simulink model "gm_sampleModel1802_5_sub"  (R2023a)
settings: Solver=VariableStepAuto  StartTime=0.0  StopTime=10.0  RelTol=1e-3
libraries: simulink x1
settings Model: Creator=user1  LastModifiedBy=user1
settings OptimizationCC: BlockReduction=off  ConditionallyExecuteInputs=off
settings DebuggingCC: InheritedTsInSrcMsg=none

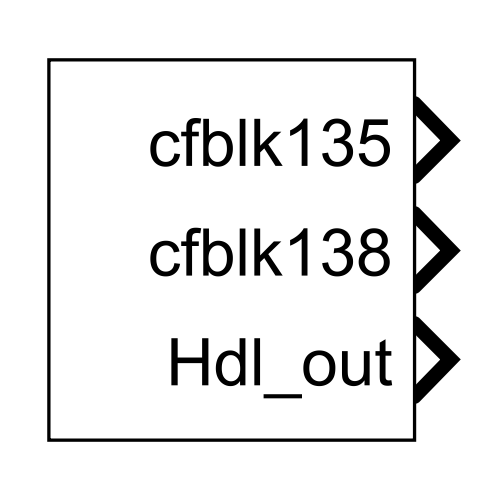
[thumbnail: Simulink's stored preview of the top-level diagram]
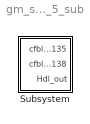
== system gm_sampleModel1802_5_sub ==
  Subsystem : Subsystem

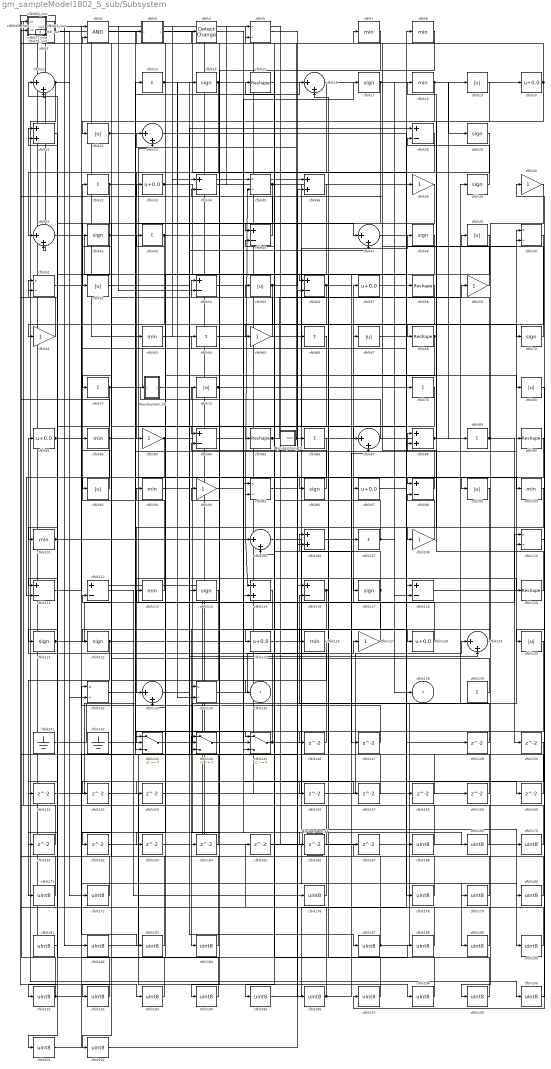
== system gm_sampleModel1802_5_sub/Subsystem ==
  Mysubsystem_19 : Subsystem
  Mysubsystem_30 : Subsystem
  Mysubsystem_45 : Subsystem
  cfblk1 : Subsystem  mask(Compare To Zero){relop=<=, OutDataTypeStr=uint8, ZeroCross=on}
      mask prompts: relop "Simulink:masks:Operator_MP"; OutDataTypeStr "Simulink:masks:OutputDataType_MP"; ZeroCross "Simulink:masks:EnableZerocrossingDetection_MP"
      mask help: Simulink:masks:CompareToZero_MD
      mask init:
      | OutDataTypeStr = 'uint8';
      | ZeroCross = 'on';
      | blkName = 'sampleModel1802_5_sub/Subsystem/cfblk1';
      | relop = '<=';
      | setValue = 'fixdt(0, 8)';
      mask TypeOptions relop: == | ~= | < | <= | >= | >
      mask TypeOptions OutDataTypeStr: Simulink:masks:uint8 | Simulink:masks:boolean
      mask Callback ZeroCross: sl('zeroCrossEnable', gcbh);
      mask Display: disp([relop,' 0'])
  cfblk{7..8,18,63,82,93,100..101,113,126} (10 alike) : MinMax  OutDataTypeStr=uint8
  cfblk103_inst : Subsystem
  cfblk{11,16,23,41,47,87,105,129,133} (9 alike) : Sum  Inputs=|++  OutDataTypeStr=uint8
  cfblk{21,36,88,106,115} (5 alike) : Sum  OutDataTypeStr=uint8
  cfblk{13,32,43,64,66,72,78,86,89,107} (10 alike) : Sum  Inputs=+  OutDataTypeStr=uint8
  cfblk{38,40,59,61,65,83,94,108,127} (9 alike) : Gain  OutDataTypeStr=uint8
  cfblk{5,35,50..51,95,110,132,134} (8 alike) : Product  Inputs=*/  OutDataTypeStr=uint8  RndMeth=Zero  SaturateOnIntegerOverflow=on
  cfblk{28,34,45,54,56,84,98,111..112,116,118} (11 alike) : Sum  Inputs=+-  OutDataTypeStr=uint8
  cfblk{14,17,29,39,42,48,70,96,114,117,121..122} (12 alike) : Signum
  cfblk{15,58,68,85,90,120} (6 alike) : Reshape
  cfblk{20,33,57,81,97,125,128} (7 alike) : Bias  Bias=0.0  SaturateOnIntegerOverflow=off
  cfblk{19,22,49,52,55,67,74,80,92,99,130} (11 alike) : Abs  OutDataTypeStr=uint8  SaturateOnIntegerOverflow=off
  cfblk131_inst : Subsystem
  cfblk139 : Constant  OutDataTypeStr=uint8  SampleTime=-1
  cfblk141 : Ground
  cfblk142 : Ground
  cfblk143 : Switch  OutDataTypeStr=uint8  SaturateOnIntegerOverflow=off  InputSameDT=off
  cfblk144 : Switch  OutDataTypeStr=uint8  SaturateOnIntegerOverflow=off  InputSameDT=off
  cfblk145 : Switch  OutDataTypeStr=uint8  SaturateOnIntegerOverflow=off  InputSameDT=off
  cfblk{146..147,149..153,156..167} (19 alike) : Delay  SampleTime=1
  cfblk{168..172,176,178..184,187..202} (29 alike) : DataTypeConversion  OutDataTypeStr=uint8  SaturateOnIntegerOverflow=off  RndMeth=Floor
  cfblk2 : Logic  AllPortsSameDT=off  OutDataTypeStr=boolean
  cfblk24_inst : Subsystem
  cfblk25_inst : Subsystem
  cfblk3 : Subsystem  mask(Compare To Constant){relop=<=, const=double(3), OutDataTypeStr=uint8, ZeroCross=on}
      mask prompts: relop "Simulink:masks:Operator_MP"; const "Simulink:masks:ConstantValue_MP"; OutDataTypeStr "Simulink:masks:OutputDataType_MP"; ZeroCross "Simulink:masks:EnableZerocrossingDetection_MP"
      mask help: Simulink:masks:CompareToConstant_MD
      mask init:
      | OutDataTypeStr = 'uint8';
      | ZeroCross = 'on';
      | blkName = 'sampleModel1802_5_sub/Subsystem/cfblk3';
      | const = double(3);
      | const_str = '3.0';
      | const_val = double(3);
      | relop = '<=';
      | setValue = 'fixdt(0, 8)';
      | str = '<= 3';
      mask TypeOptions relop: == | ~= | < | <= | >= | >
      mask TypeOptions OutDataTypeStr: Simulink:masks:uint8 | Simulink:masks:boolean
      mask Callback ZeroCross: sl('zeroCrossEnable', gcbh);
      mask Display: disp(str)
  cfblk4 : simulink/Logic and Bit Operations/Detect Change  vinit=0  OutDataTypeStr=uint8
      settings: LibrarySourceBlock=|
      | hdlsllib/Logic and Bit
      | Operations/Detect
      | Change
  cfblk53_inst : Subsystem
  cfblk60_inst : Subsystem
  cfblk69_inst : Subsystem
  cfblk71_inst : Subsystem
  cfblk75_inst : Subsystem
  cfblk135 : Outport  OutDataTypeStr=uint8  SampleTime=1  VectorParamsAs1DForOutWhenUnconnected=off
  cfblk138 : Outport  Port=2  OutDataTypeStr=uint8  SampleTime=1  VectorParamsAs1DForOutWhenUnconnected=off
  Hdl_out : Outport  Port=3  OutDataTypeStr=uint8
  wires:
  Mysubsystem_19/1(Out1) -> cfblk25_inst/1(in1), cfblk23/1
  Mysubsystem_30/1(Out1) -> Mysubsystem_45/1(In1)
  Mysubsystem_45/1(Out1) -> cfblk112/1
  cfblk1/1(y) -> cfblk193/1, cfblk172/1
  cfblk100/1 -> cfblk133/1
  cfblk101/1 -> cfblk115/1, cfblk35/2
  cfblk103_inst/1(out1) -> cfblk182/1
  cfblk105/1 -> cfblk190/1
  cfblk106/1 -> cfblk57/1
  cfblk107/1 -> cfblk15/1, cfblk138/1
  cfblk108/1 -> cfblk98/2
  cfblk11/1 -> cfblk200/1, cfblk132/2
  cfblk110/1 -> cfblk197/1
  cfblk111/1 -> cfblk64/1
  cfblk112/1 -> cfblk176/1
  cfblk113/1 -> cfblk32/1
  cfblk114/1 -> cfblk202/1
  cfblk115/1 -> cfblk162/1
  cfblk116/1 -> cfblk16/2, cfblk125/1
  cfblk117/1 -> cfblk74/1, cfblk184/1
  cfblk118/1 -> cfblk50/1
  cfblk120/1 -> cfblk88/1
  cfblk121/1 -> cfblk97/1, cfblk23/2
  cfblk122/1 -> cfblk171/1, cfblk17/1
  cfblk125/1 -> cfblk48/1
  cfblk126/1 -> cfblk134/1
  cfblk127/1 -> cfblk54/1
  cfblk128/1 -> cfblk113/1
  cfblk129/1 -> cfblk122/1
  cfblk13/1 -> cfblk114/1, cfblk134/2
  cfblk130/1 -> cfblk143/2
  cfblk131_inst/1(out1) -> cfblk89/1
  cfblk132/1 -> cfblk145/1
  cfblk133/1 -> cfblk129/2
  cfblk134/1 -> cfblk127/1
  cfblk139/1 -> cfblk82/1
  cfblk14/1 -> cfblk68/1, cfblk83/1, cfblk164/1
  cfblk141/1 -> cfblk90/1
  cfblk142/1 -> cfblk13/1
  cfblk143/1 -> cfblk110/2
  cfblk144/1 -> cfblk88/2
  cfblk145/1 -> cfblk81/1, cfblk107/1
  cfblk146/1 -> cfblk11/1
  cfblk147/1 -> cfblk132/1
  cfblk149/1 -> cfblk116/2
  cfblk15/1 -> cfblk45/1
  cfblk150/1 -> cfblk192/1
  cfblk151/1 -> cfblk16/1
  cfblk152/1 -> cfblk198/1
  cfblk153/1 -> cfblk110/1
  cfblk156/1 -> cfblk129/1
  cfblk157/1 -> cfblk133/2
  cfblk158/1 -> cfblk144/1
  cfblk159/1 -> cfblk45/2
  cfblk16/1 -> cfblk85/1
  cfblk160/1 -> cfblk2/2
  cfblk161/1 -> cfblk69_inst/2(in2)
  cfblk162/1 -> cfblk34/1
  cfblk163/1 -> cfblk180/1
  cfblk164/1 -> cfblk131_inst/2(in2)
  cfblk165/1 -> cfblk189/1
  cfblk166/1 -> cfblk24_inst/2(in2)
  cfblk167/1 -> cfblk1/1(u)
  cfblk168/1 -> cfblk55/1
  cfblk169/1 -> cfblk3/1(u)
  cfblk17/1 -> cfblk121/1, cfblk118/2
  cfblk170/1 -> cfblk94/1
  cfblk171/1 -> cfblk60_inst/1(in1)
  cfblk172/1 -> cfblk60_inst/2(in2)
  cfblk176/1 -> cfblk25_inst/2(in2)
  cfblk178/1 -> cfblk112/2
  cfblk179/1 -> cfblk24_inst/1(in1)
  cfblk18/1 -> cfblk29/1, cfblk105/2
  cfblk180/1 -> cfblk51/1
  cfblk181/1 -> cfblk51/2
  cfblk182/1 -> cfblk116/1
  cfblk183/1 -> cfblk103_inst/1(in1)
  cfblk184/1 -> cfblk103_inst/2(in2)
  cfblk187/1 -> cfblk39/1, cfblk167/1
  cfblk188/1 -> cfblk93/1
  cfblk189/1 -> cfblk71_inst/1(in1)
  cfblk19/1 -> cfblk108/1
  cfblk190/1 -> cfblk165/1
  cfblk191/1 -> cfblk71_inst/2(in2), cfblk188/1, cfblk144/3
  cfblk192/1 -> cfblk21/1
  cfblk193/1 -> cfblk21/2
  cfblk194/1 -> cfblk33/1
  cfblk195/1 -> cfblk78/1
  cfblk196/1 -> cfblk87/2, cfblk43/1
  cfblk197/1 -> cfblk5/1
  cfblk198/1 -> cfblk5/2
  cfblk199/1 -> cfblk106/1
  cfblk2/1 -> cfblk117/1
  cfblk20/1 -> cfblk22/1, cfblk131_inst/1(in1)
  cfblk200/1 -> cfblk40/1
  cfblk201/1 -> cfblk143/1
  cfblk202/1 -> cfblk86/1
  cfblk21/1 -> cfblk191/1
  cfblk22/1 -> cfblk87/1, cfblk105/1
  cfblk23/1 -> cfblk178/1
  cfblk24_inst/1(out1) -> cfblk11/2, cfblk63/1
  cfblk25_inst/1(out1) -> cfblk54/2, cfblk20/1
  cfblk28/1 -> cfblk61/1
  cfblk29/1 -> cfblk41/1
  cfblk3/1(y) -> cfblk168/1
  cfblk32/1 -> cfblk98/1, cfblk52/1
  cfblk33/1 -> cfblk28/1, cfblk14/1, cfblk118/1
  cfblk34/1 -> cfblk128/1
  cfblk35/1 -> cfblk70/1, cfblk111/1, cfblk158/1
  cfblk36/1 -> cfblk153/1
  cfblk38/1 -> cfblk72/1
  cfblk39/1 -> cfblk18/1
  cfblk4/1 -> cfblk56/1
  cfblk40/1 -> cfblk199/1
  cfblk41/1 -> cfblk147/1
  cfblk42/1 -> cfblk75_inst/2(in2), cfblk47/1, cfblk101/1
  cfblk43/1 -> cfblk169/1, cfblk151/1
  cfblk45/1 -> cfblk69_inst/1(in1)
  cfblk47/1 -> cfblk99/1
  cfblk48/1 -> cfblk96/1
  cfblk49/1 -> cfblk95/2
  cfblk5/1 -> cfblk196/1
  cfblk50/1 -> cfblk65/1
  cfblk51/1 -> cfblk179/1
  cfblk52/1 -> cfblk100/1
  cfblk53_inst/1(out1) -> cfblk159/1
  cfblk54/1 -> cfblk120/1
  cfblk55/1 -> cfblk36/2, cfblk152/1
  cfblk56/1 -> cfblk80/1, cfblk144/2
  cfblk57/1 -> cfblk58/1
  cfblk58/1 -> cfblk146/1
  cfblk59/1 -> cfblk34/2
  cfblk60_inst/1(out1) -> cfblk170/1
  cfblk61/1 -> cfblk75_inst/1(in1)
  cfblk63/1 -> cfblk47/2
  cfblk64/1 -> cfblk95/1
  cfblk65/1 -> cfblk42/1
  cfblk66/1 -> cfblk92/1
  cfblk67/1 -> cfblk160/1
  cfblk68/1 -> cfblk115/2, cfblk163/1
  cfblk69_inst/1(out1) -> cfblk41/2, cfblk66/1
  cfblk7/1 -> cfblk195/1
  cfblk70/1 -> cfblk53_inst/1(in1)
  cfblk71_inst/1(out1) -> cfblk36/1, cfblk181/1
  cfblk72/1 -> cfblk35/1, cfblk161/1, cfblk8/1
  cfblk74/1 -> cfblk56/2, cfblk49/1
  cfblk75_inst/1(out1) -> cfblk38/1
  cfblk78/1 -> cfblk194/1
  cfblk8/1 -> cfblk84/1
  cfblk80/1 -> cfblk130/1
  cfblk81/1 -> cfblk183/1, cfblk166/1
  cfblk82/1 -> cfblk53_inst/2(in2), cfblk145/3, cfblk111/2
  cfblk83/1 -> cfblk143/3, cfblk106/2
  cfblk84/1 -> cfblk157/1
  cfblk85/1 -> cfblk59/1, cfblk135/1
  cfblk86/1 -> cfblk201/1
  cfblk87/1 -> Mysubsystem_30/1(In1)
  cfblk88/1 -> cfblk28/2, cfblk19/1, cfblk50/2
  cfblk89/1 -> cfblk150/1, cfblk4/1
  cfblk90/1 -> cfblk145/2
  cfblk92/1 -> cfblk2/1
  cfblk93/1 -> cfblk187/1
  cfblk94/1 -> cfblk126/1
  cfblk95/1 -> cfblk67/1
  cfblk96/1 -> cfblk84/2
  cfblk97/1 -> cfblk149/1
  cfblk98/1 -> cfblk7/1
  cfblk99/1 -> cfblk156/1

== system gm_sampleModel1802_5_sub/Subsystem/Mysubsystem_19 ==
  cfblk140 : Subsystem  mask(Counter Limited){uplimit=double(7), tsamp=double(-1)}
      mask prompts: uplimit "Simulink:masks:UpperLimit_MP"; tsamp "Simulink:masks:SampleTime_MP"
      mask help: Simulink:masks:CounterLimited_MD
      mask init:
      | nbits = double(8);
      | tsamp = double(-1);
      | uplimit = double(7);
  cfblk31 : Bias  Bias=0.0  SaturateOnIntegerOverflow=off
  Out1 : Outport  SampleTime=1
  wires:
  cfblk140/1(y) -> cfblk31/1
  cfblk31/1 -> Out1/1

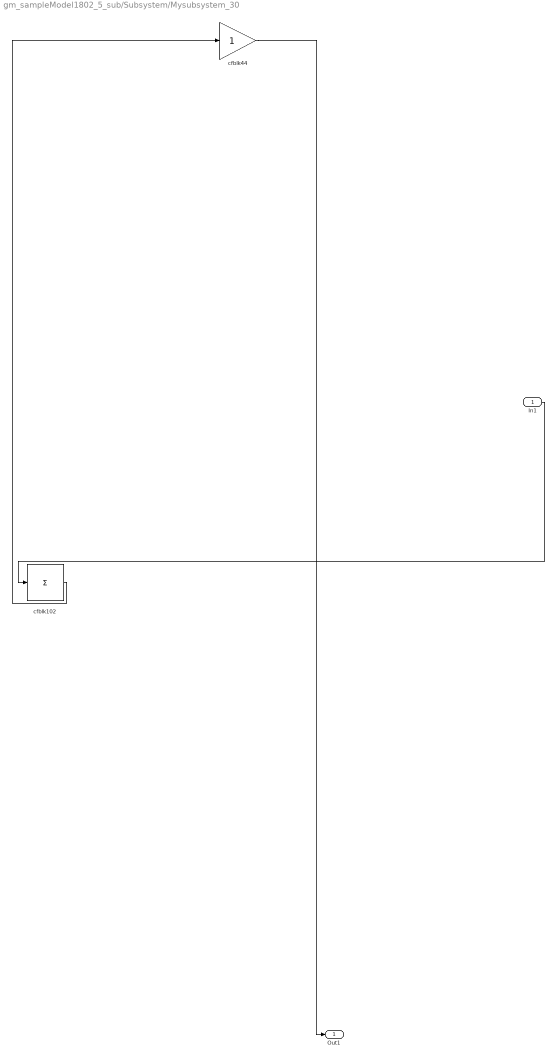
== system gm_sampleModel1802_5_sub/Subsystem/Mysubsystem_30 ==
  In1 : Inport  OutDataTypeStr=uint8  PortDimensions=1  SampleTime=1
  cfblk102 : Sum  Inputs=+
  cfblk44 : Gain
  Out1 : Outport  SampleTime=1
  wires:
  In1/1 -> cfblk102/1
  cfblk102/1 -> cfblk44/1
  cfblk44/1 -> Out1/1

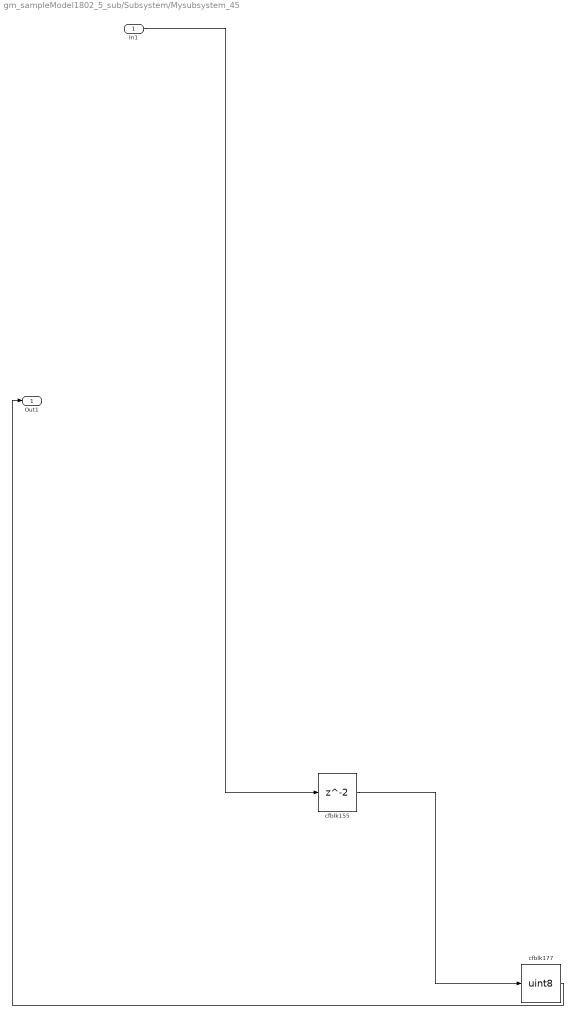
== system gm_sampleModel1802_5_sub/Subsystem/Mysubsystem_45 ==
  In1 : Inport  OutDataTypeStr=fixdt(0, 16, 7)  PortDimensions=1  SampleTime=1
  cfblk155 : Delay  SampleTime=1
  cfblk177 : DataTypeConversion  OutDataTypeStr=uint8  SaturateOnIntegerOverflow=off  RndMeth=Floor
  Out1 : Outport  SampleTime=1
  wires:
  In1/1 -> cfblk155/1
  cfblk155/1 -> cfblk177/1
  cfblk177/1 -> Out1/1

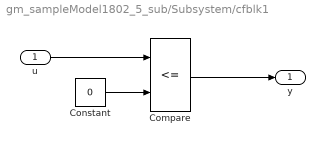
== system gm_sampleModel1802_5_sub/Subsystem/cfblk1 ==
  u : Inport  OutDataTypeStr=uint8  SampleTime=1
  Compare : RelationalOperator  Operator=<=  OutDataTypeStr=fixdt(0, 8)
  Constant : Constant  DisableCoverage=on  Value=0  OutDataTypeStr=Inherit: Inherit via back propagation  SampleTime=-1  PreserveConstantTs=on
  y : Outport  SampleTime=1
  wires:
  u/1 -> Compare/1
  Compare/1 -> y/1
  Constant/1 -> Compare/2

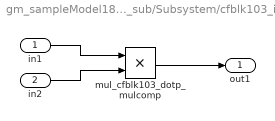
== system gm_sampleModel1802_5_sub/Subsystem/cfblk103_inst ==
  in1 : Inport  OutDataTypeStr=uint8  SampleTime=1
  in2 : Inport  Port=2  OutDataTypeStr=uint8  SampleTime=1
  mul_cfblk103_dotp_mulcomp : Product  Inputs=**  OutDataTypeStr=uint8  SampleTime=1
  out1 : Outport  OutDataTypeStr=uint8  SampleTime=1
  wires:
  in1/1 -> mul_cfblk103_dotp_mulcomp/1
  in2/1 -> mul_cfblk103_dotp_mulcomp/2
  mul_cfblk103_dotp_mulcomp/1 -> out1/1

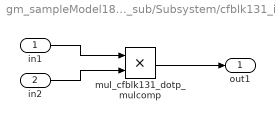
== system gm_sampleModel1802_5_sub/Subsystem/cfblk131_inst ==
  in1 : Inport  OutDataTypeStr=uint8  SampleTime=1
  in2 : Inport  Port=2  OutDataTypeStr=uint8  SampleTime=1
  mul_cfblk131_dotp_mulcomp : Product  Inputs=**  OutDataTypeStr=uint8  SampleTime=1
  out1 : Outport  OutDataTypeStr=uint8  SampleTime=1
  wires:
  in1/1 -> mul_cfblk131_dotp_mulcomp/1
  in2/1 -> mul_cfblk131_dotp_mulcomp/2
  mul_cfblk131_dotp_mulcomp/1 -> out1/1

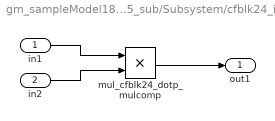
== system gm_sampleModel1802_5_sub/Subsystem/cfblk24_inst ==
  in1 : Inport  OutDataTypeStr=uint8  SampleTime=1
  in2 : Inport  Port=2  OutDataTypeStr=uint8  SampleTime=1
  mul_cfblk24_dotp_mulcomp : Product  Inputs=**  OutDataTypeStr=uint8  SampleTime=1
  out1 : Outport  OutDataTypeStr=uint8  SampleTime=1
  wires:
  in1/1 -> mul_cfblk24_dotp_mulcomp/1
  in2/1 -> mul_cfblk24_dotp_mulcomp/2
  mul_cfblk24_dotp_mulcomp/1 -> out1/1

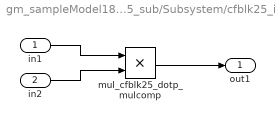
== system gm_sampleModel1802_5_sub/Subsystem/cfblk25_inst ==
  in1 : Inport  OutDataTypeStr=uint8  SampleTime=1
  in2 : Inport  Port=2  OutDataTypeStr=uint8  SampleTime=1
  mul_cfblk25_dotp_mulcomp : Product  Inputs=**  OutDataTypeStr=uint8  SampleTime=1
  out1 : Outport  OutDataTypeStr=uint8  SampleTime=1
  wires:
  in1/1 -> mul_cfblk25_dotp_mulcomp/1
  in2/1 -> mul_cfblk25_dotp_mulcomp/2
  mul_cfblk25_dotp_mulcomp/1 -> out1/1

== system gm_sampleModel1802_5_sub/Subsystem/cfblk3 ==
  u : Inport  OutDataTypeStr=uint8  SampleTime=1
  Compare : RelationalOperator  Operator=<=  OutDataTypeStr=fixdt(0, 8)
  Constant : Constant  DisableCoverage=on  Value=const  OutDataTypeStr=Inherit: Inherit via back propagation  SampleTime=-1
  y : Outport  SampleTime=1
  wires:
  u/1 -> Compare/1
  Compare/1 -> y/1
  Constant/1 -> Compare/2

== system gm_sampleModel1802_5_sub/Subsystem/cfblk53_inst ==
  in1 : Inport  OutDataTypeStr=uint8  SampleTime=1
  in2 : Inport  Port=2  OutDataTypeStr=uint8  SampleTime=1
  mul_cfblk53_dotp_mulcomp : Product  Inputs=**  OutDataTypeStr=uint8  SampleTime=1
  out1 : Outport  OutDataTypeStr=uint8  SampleTime=1
  wires:
  in1/1 -> mul_cfblk53_dotp_mulcomp/1
  in2/1 -> mul_cfblk53_dotp_mulcomp/2
  mul_cfblk53_dotp_mulcomp/1 -> out1/1

== system gm_sampleModel1802_5_sub/Subsystem/cfblk60_inst ==
  in1 : Inport  OutDataTypeStr=uint8  SampleTime=1
  in2 : Inport  Port=2  OutDataTypeStr=uint8  SampleTime=1
  mul_cfblk60_dotp_mulcomp : Product  Inputs=**  OutDataTypeStr=uint8  SampleTime=1
  out1 : Outport  OutDataTypeStr=uint8  SampleTime=1
  wires:
  in1/1 -> mul_cfblk60_dotp_mulcomp/1
  in2/1 -> mul_cfblk60_dotp_mulcomp/2
  mul_cfblk60_dotp_mulcomp/1 -> out1/1

== system gm_sampleModel1802_5_sub/Subsystem/cfblk69_inst ==
  in1 : Inport  OutDataTypeStr=uint8  SampleTime=1
  in2 : Inport  Port=2  OutDataTypeStr=uint8  SampleTime=1
  mul_cfblk69_dotp_mulcomp : Product  Inputs=**  OutDataTypeStr=uint8  SampleTime=1
  out1 : Outport  OutDataTypeStr=uint8  SampleTime=1
  wires:
  in1/1 -> mul_cfblk69_dotp_mulcomp/1
  in2/1 -> mul_cfblk69_dotp_mulcomp/2
  mul_cfblk69_dotp_mulcomp/1 -> out1/1

== system gm_sampleModel1802_5_sub/Subsystem/cfblk71_inst ==
  in1 : Inport  OutDataTypeStr=uint8  SampleTime=1
  in2 : Inport  Port=2  OutDataTypeStr=uint8  SampleTime=1
  mul_cfblk71_dotp_mulcomp : Product  Inputs=**  OutDataTypeStr=uint8  SampleTime=1
  out1 : Outport  OutDataTypeStr=uint8  SampleTime=1
  wires:
  in1/1 -> mul_cfblk71_dotp_mulcomp/1
  in2/1 -> mul_cfblk71_dotp_mulcomp/2
  mul_cfblk71_dotp_mulcomp/1 -> out1/1

== system gm_sampleModel1802_5_sub/Subsystem/cfblk75_inst ==
  in1 : Inport  OutDataTypeStr=uint8  SampleTime=1
  in2 : Inport  Port=2  OutDataTypeStr=uint8  SampleTime=1
  mul_cfblk75_dotp_mulcomp : Product  Inputs=**  OutDataTypeStr=uint8  SampleTime=1
  out1 : Outport  OutDataTypeStr=uint8  SampleTime=1
  wires:
  in1/1 -> mul_cfblk75_dotp_mulcomp/1
  in2/1 -> mul_cfblk75_dotp_mulcomp/2
  mul_cfblk75_dotp_mulcomp/1 -> out1/1

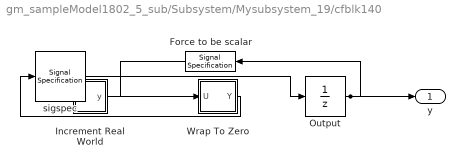
== system gm_sampleModel1802_5_sub/Subsystem/Mysubsystem_19/cfblk140 ==
  Force to be scalar : SignalSpecification  DisableCoverage=on  Dimensions=1
  Increment Real World : Subsystem  mask(Real World Value Increment){}
      mask help: Simulink:masks:RealWorldValueIncrement_MD
      mask Display: disp('V++')
  Output : UnitDelay  InitialCondition=0.0  SampleTime=tsamp  HasFrameUpgradeWarning=on
  Wrap To Zero : Subsystem  mask(Wrap To Zero){Threshold=double(7)}
      mask prompts: Threshold "Simulink:masks:Threshold_MP"
      mask help: Simulink:masks:WrapToZero_MD
  sigspec : SignalSpecification  OutDataTypeStr=uint8  Dimensions=1
  y : Outport  SampleTime=1
  wires:
  Force to be scalar/1 -> Increment Real World/1(u)
  Increment Real World/1(y) -> Wrap To Zero/1(U)
  Output/1 -> Force to be scalar/1, y/1
  Wrap To Zero/1(Y) -> sigspec/1
  sigspec/1 -> Output/1

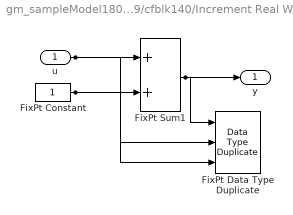
== system gm_sampleModel1802_5_sub/Subsystem/Mysubsystem_19/cfblk140/Increment Real World ==
  u : Inport  OutDataTypeStr=uint8  SampleTime=1
  FixPt Constant : Constant  DisableCoverage=on  OutDataTypeStr=Inherit: Inherit via back propagation  SampleTime=-1
  FixPt Data Type Duplicate : DataTypeDuplicate  DisableCoverage=on  NumInputPorts=3
  FixPt Sum1 : Sum  InputSameDT=on  OutDataTypeStr=Inherit: Inherit via back propagation  LockScale=on
  y : Outport  SampleTime=1
  wires:
  u/1 -> FixPt Sum1/1, FixPt Data Type Duplicate/2
  FixPt Constant/1 -> FixPt Sum1/2, FixPt Data Type Duplicate/3
  FixPt Sum1/1 -> FixPt Data Type Duplicate/1, y/1

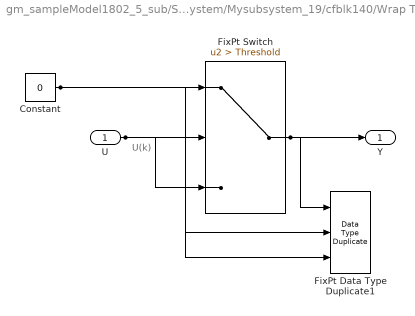
== system gm_sampleModel1802_5_sub/Subsystem/Mysubsystem_19/cfblk140/Wrap To Zero ==
  note: U(k)
  U : Inport  OutDataTypeStr=uint8  SampleTime=1
  Constant : Constant  DisableCoverage=on  Value=0  OutDataTypeStr=Inherit: Inherit via back propagation  SampleTime=-1
  FixPt Data Type Duplicate1 : DataTypeDuplicate  DisableCoverage=on  NumInputPorts=3
  FixPt Switch : Switch  Criteria=u2 > Threshold  Threshold=Threshold  OutDataTypeStr=Inherit: Inherit via back propagation  ZeroCross=off  SaturateOnIntegerOverflow=off  InputSameDT=off
  Y : Outport  SampleTime=1
  wires:
  U/1 -> FixPt Switch/3, FixPt Switch/2, FixPt Data Type Duplicate1/2
  Constant/1 -> FixPt Switch/1, FixPt Data Type Duplicate1/3
  FixPt Switch/1 -> FixPt Data Type Duplicate1/1, Y/1
